simulink model "levitate_model"  (R2023b)
settings: Solver=VariableStepAuto  StartTime=0.0  StopTime=100  RelTol=1e-3
values from neighbouring files (symbols this model uses):
  g = 9.81    [levitate_param.m]
  K = 0.005    [levitate_param.m]
  L = 0.01    [levitate_param.m]
  m = 0.05    [levitate_param.m]
  R = 5    [levitate_param.m]
  u_0 = R* sqrt(m*g*x_d^2/K)    [levitate_param.m]
  x_0 = 0.03    [levitate_param.m]
  x_d = 0.05    [levitate_param.m]
libraries: simulink x1, fuzblock x1, slpidlib x1
settings Model: Creator=zhy  LastModifiedBy=zhy

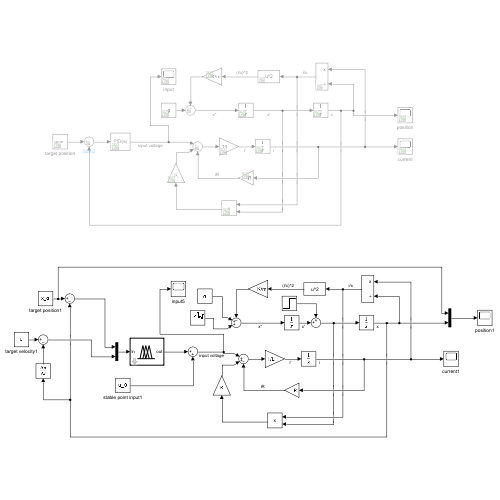
[thumbnail: Simulink's stored preview of the top-level diagram]
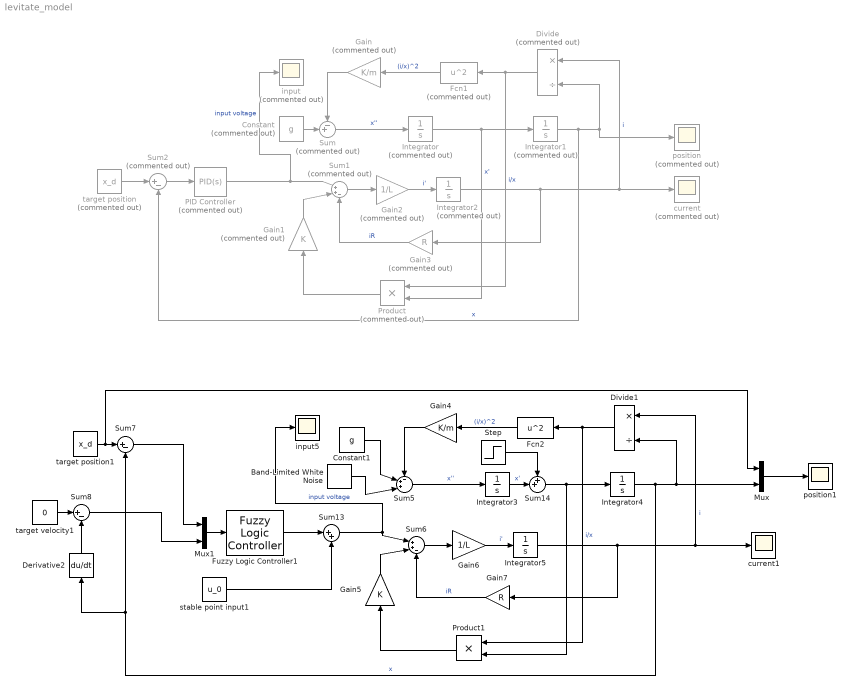
== system levitate_model ==
  Band-Limited White Noise : simulink/Sources/Band-Limited White Noise  Cov=[0.05]  Ts=0.01  seed=[23341]
  Constant : Constant  Commented=on  Value=g
  Constant1 : Constant  Value=g
  Derivative2 : Derivative
  Divide : Product  Commented=on  Inputs=*/
  Divide1 : Product  Inputs=*/
  Fcn1 : Fcn  Commented=on  Expr=u^2
  Fcn2 : Fcn  Expr=u^2
  Fuzzy Logic Controller1 : fuzblock/Fuzzy Logic  Controller  FIS='levitate_controller.fis'  OutputSampleNumber=101  DataType=double  FuzzifiedInputs=off  RuleFiringStrengths=off  RuleOutputs=off  AggregatedOutputs=off  SimulateUsing=Interpreted execution  OutOfRangeInputValueMessage=warning  NoRuleFiredMessage=warning  EmptyOutputFuzzySetMessage=warning
  Gain : Gain  Commented=on  Gain=K/m
  Gain1 : Gain  Commented=on  Gain=K
  Gain2 : Gain  Commented=on  Gain=1/L
  Gain3 : Gain  Commented=on  Gain=R
  Gain4 : Gain  Gain=K/m
  Gain5 : Gain  Gain=K
  Gain6 : Gain  Gain=1/L
  Gain7 : Gain  Gain=R
  Integrator : Integrator  Commented=on
  Integrator1 : Integrator  Commented=on  InitialCondition=x_0
  Integrator2 : Integrator  Commented=on
  Integrator3 : Integrator
  Integrator4 : Integrator  InitialCondition=x_0
  Integrator5 : Integrator
  Mux : Mux  Inputs=2
  Mux1 : Mux  Inputs=2
  PID Controller : slpidlib/PID Controller  Commented=on  Controller=PID  Form=Parallel  TimeDomain=Continuous-time  UseExternalTs=off  SampleTime=-1  IntegratorMethod=Forward Euler  FilterMethod=Forward Euler  ControllerParametersSource=internal  P=72  I=1.5  UseKiTs=on  D=0.2  N=100  UseFilter=on  TunerSelectOption=Transfer Function Based (PID Tuner App)  InitialConditionSource=internal  InitialConditionForIntegrator=0  InitialConditionForFilter=0  DifferentiatorICPrevScaledInput=0  ExternalReset=none  TrackingMode=off  Kt=1  LimitOutput=off  SatLimitsSource=internal  UpperSaturationLimit=inf  LowerSaturationLimit=-inf  LinearizeAsGain=on  AntiWindupMode=none  Kb=1  LimitIntegrator=off  UpperIntegratorSaturationLimit=inf  LowerIntegratorSaturationLimit=-inf  POutMin=[]  POutMax=[]  IOutMin=[]  IOutMax=[]  DOutMin=[]  DOutMax=[]  NOutMin=[]  NOutMax=[]  SumOutMin=[]  SumOutMax=[]  SaturationOutMin=[]  SaturationOutMax=[]  PParamMin=[]  PParamMax=[]  IParamMin=[]  IParamMax=[]  DParamMin=[]  DParamMax=[]  NParamMin=[]  NParamMax=[]  KbParamMin=[]  KbParamMax=[]  KtParamMin=[]  KtParamMax=[]  KbOutMin=[]  KbOutMax=[]  KtOutMin=[]  KtOutMax=[]  IntegratorOutMin=[]  IntegratorOutMax=[]  FilterOutMin=[]  FilterOutMax=[]  SumI1OutMin=[]  SumI1OutMax=[]  SumI2OutMin=[]  SumI2OutMax=[]  SumI3OutMin=[]  SumI3OutMax=[]  SumI4OutMin=[]  SumI4OutMax=[]  SumDOutMin=[]  SumDOutMax=[]  DifferentiatorOutMin=[]  DifferentiatorOutMax=[]  FilterDiffOutCoefMin=[]  FilterDiffOutCoefMax=[]  ReciprocalOutMin=[]  ReciprocalOutMax=[]  SumDenOutMin=[]  SumDenOutMax=[]  SumNumOutMin=[]  SumNumOutMax=[]  DivideOutMin=[]  DivideOutMax=[]  UdiffTsProdOutMin=[]  UdiffTsProdOutMax=[]  NTsProdOutMin=[]  NTsProdOutMax=[]  UintegralTsProdOutMin=[]  UintegralTsProdOutMax=[]  UngainTsProdOutMin=[]  UngainTsProdOutMax=[]  ClampingZeroOutDataTypeStr=Inherit: Inherit via back propagation  ClampingZeroOutMin=[]  ClampingZeroOutMax=[]  FilterDenConstantOutDataTypeStr=Inherit: Inherit via back propagation  FilterDenConstantOutMin=[]  FilterDenConstantOutMax=[]  PCopyOutDataTypeStr=Inherit: Inherit via back propagation  PCopyOutMin=[]  PCopyOutMax=[]  NCopyOutDataTypeStr=Inherit: Inherit via back propagation  NCopyOutMin=[]  NCopyOutMax=[]  IntegratorContinuousStateAttributes=''  IntegratorStateMustResolveToSignalObject=off  IntegratorRTWStateStorageClass=Auto  FilterContinuousStateAttributes=''  FilterStateMustResolveToSignalObject=off  FilterRTWStateStorageClass=Auto  ParallelPVariant=InternalParameters  IdealPVariant=Disabled  IVariant=InternalParameters  DVariant=InternalParameters  IntegratorVariant=Continuous  SatVariant=Disabled  AWVariant=Passthrough  PCopyVariant=Disabled  TRVariant=Disabled  FdbkBlocksVariant=Forward  IdealPFdbkVariant=Disabled  SatFdbkVariant=Disabled  DerivativeFilterVariant=ContFilter  NVariant=InternalParameters  NCopyVariant=Disabled  FilterICVariant=InternalICsFilter  IntegratorICVariant=InternalICs  ExternalResetVariant=Disabled  TRSumVariant=Passthrough  SumFdbkVariant=Disabled  SumVariant=Sum_PID  TsampFilterVariant=InternalTs  TsampNgainVariant=Passthrough  TsampIntegralVariant=Disabled_SignalSpec  ExternalSaturationOutDataTypeStr=Inherit: Same as second input
  Product : Product  Commented=on
  Product1 : Product
  Step : Step  Time=0.8  After=0.5  SampleTime=0
  Sum : Sum  Commented=on  Inputs=-+|
  Sum1 : Sum  Commented=on  Inputs=|++-
  Sum13 : Sum  Inputs=|++
  Sum14 : Sum  Inputs=++|
  Sum2 : Sum  Commented=on  Inputs=|+-
  Sum5 : Sum  Inputs=-++|
  Sum6 : Sum  Inputs=|++-
  Sum7 : Sum  Inputs=|+-
  Sum8 : Sum  Inputs=|+-
  current : Scope  Commented=on
  current1 : Scope
  input : Scope  Commented=on
  input5 : Scope
  position : Scope  Commented=on
  position1 : Scope
  stable point input1 : Constant  Value=u_0
  target position : Constant  Commented=on  Value=x_d
  target position1 : Constant  Value=x_d
  target velocity1 : Constant  Value=0
  wires:
  Integrator/1 -> Product/2, Integrator1/1  "x'"
  Sum/1 -> Integrator/1  "x''"
  Constant/1 -> Sum/2
  Divide/1 -> Product/1, Fcn1/1  "i/x"
  Gain/1 -> Sum/1
  Fcn1/1 -> Gain/1  "(i/x)^2"
  Integrator2/1 -> Gain3/1, Divide/1, current/1  "i"
  Integrator1/1 -> Sum2/2, position/1, Divide/2  "x"
  Gain1/1 -> Sum1/2
  Sum1/1 -> Gain2/1
  Gain2/1 -> Integrator2/1  "i'"
  Product/1 -> Gain1/1
  Gain3/1 -> Sum1/3  "iR"
  target position/1 -> Sum2/1
  Sum13/1 -> input5/1, Sum6/1  "input voltage"
  Sum8/1 -> Mux1/2
  Gain6/1 -> Integrator5/1  "i'"
  target velocity1/1 -> Sum8/1
  Sum7/1 -> Mux1/1
  Fcn2/1 -> Gain4/1  "(i/x)^2"
  Sum6/1 -> Gain6/1
  Mux1/1 -> Fuzzy Logic Controller1/1
  Gain7/1 -> Sum6/3  "iR"
  Gain5/1 -> Sum6/2
  Integrator4/1 -> Derivative2/1, Sum7/2, Divide1/2, Mux/2  "x"
  Gain4/1 -> Sum5/1
  Divide1/1 -> Product1/1, Fcn2/1  "i/x"
  Product1/1 -> Gain5/1
  Integrator5/1 -> Gain7/1, Divide1/1, current1/1  "i"
  Sum5/1 -> Integrator3/1  "x''"
  Derivative2/1 -> Sum8/2
  target position1/1 -> Mux/1, Sum7/1
  Constant1/1 -> Sum5/2
  Fuzzy Logic Controller1/1 -> Sum13/1
  stable point input1/1 -> Sum13/2
  Band-Limited White Noise/1 -> Sum5/3
  Sum14/1 -> Product1/2, Integrator4/1
  Step/1 -> Sum14/1
  Integrator3/1 -> Sum14/2  "x'"
  Sum2/1 -> PID Controller/1
  Mux/1 -> position1/1
  PID Controller/1 -> input/1, Sum1/1  "input voltage"
